simulink model "Scenario_2"  (R2025b)
settings: Solver=VariableStepAuto  StartTime=0.0  StopTime=20.0  RelTol=1e-3
libraries: SignalEditorBlockLib x2
settings Model: Creator=danai  LastModifiedBy=danai

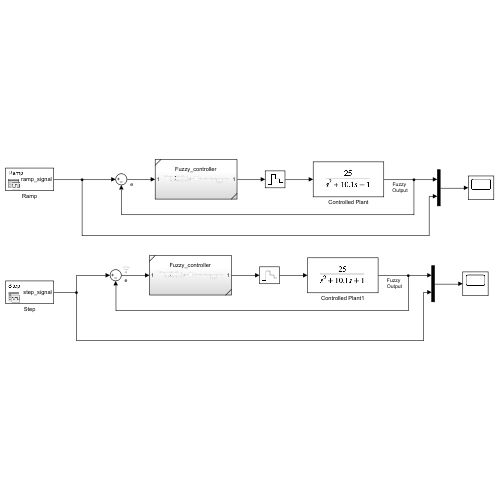
[thumbnail: Simulink's stored preview of the top-level diagram]
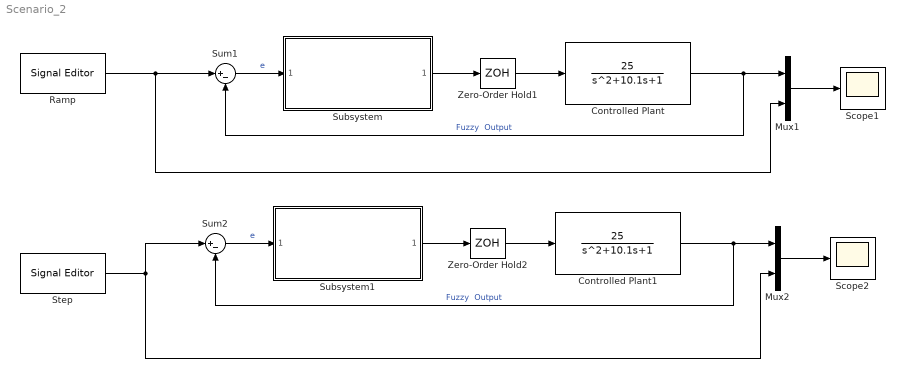
== system Scenario_2 ==
  Controlled Plant : TransferFcn  Numerator=[25]  Denominator=[1 10.1 1]
  Controlled Plant1 : TransferFcn  Numerator=[25]  Denominator=[1 10.1 1]
  Mux1 : Mux  Inputs=2
  Mux2 : Mux  Inputs=2
  Ramp : SignalEditorBlockLib/Signal Editor  FileName=signals.mat  ActiveScenario=Ramp  ActiveSignal=ramp_signal  IsBus=off  OutputBusObjectStr=Bus: BusObject  SampleTime=0  ZeroCross=off  OutputAfterFinalValue=Setting to zero  Unit=inherit  PreserveSignalName=on  ApplySigPropsToAllScenarios=on  ApplySigPropsToAllSignals=off  SignalPropertySource=Dialog parameters
  Scope1 : Scope
      settings: ActiveDisplayYMinimum=-7.8964112180408925  ActiveDisplayYMaximum=103.27564705951956
  Scope2 : Scope
      settings: ActiveDisplayYMinimum=-3.5810948381696477  ActiveDisplayYMaximum=79.377206724330364
  Step : SignalEditorBlockLib/Signal Editor  FileName=signals.mat  ActiveScenario=Step  ActiveSignal=step_signal  IsBus=off  OutputBusObjectStr=Bus: BusObject  SampleTime=0  Interpolate=off  ZeroCross=off  OutputAfterFinalValue=Holding final value  Unit=inherit  PreserveSignalName=on  ApplySigPropsToAllScenarios=on  ApplySigPropsToAllSignals=off  SignalPropertySource=Dialog parameters
  Subsystem : Subsystem  ReferencedSubsystem=Fuzzy_controller
  Subsystem1 : Subsystem  ReferencedSubsystem=Fuzzy_controller
  Sum1 : Sum  Inputs=|+-
  Sum2 : Sum  Inputs=|+-
  Zero-Order Hold1 : ZeroOrderHold  SampleTime=-1
  Zero-Order Hold2 : ZeroOrderHold  SampleTime=-1
  wires:
  Ramp/1 -> Mux1/2, Sum1/1
  Mux1/1 -> Scope1/1
  Zero-Order Hold1/1 -> Controlled Plant/1
  Controlled Plant/1 -> Sum1/2, Mux1/1  "Fuzzy  Output"
  Sum1/1 -> Subsystem/1  "e"
  Subsystem/1 -> Zero-Order Hold1/1
  Zero-Order Hold2/1 -> Controlled Plant1/1
  Step/1 -> Mux2/2, Sum2/1
  Mux2/1 -> Scope2/1
  Controlled Plant1/1 -> Sum2/2, Mux2/1  "Fuzzy  Output"
  Sum2/1 -> Subsystem1/1  "e"
  Subsystem1/1 -> Zero-Order Hold2/1
